simulink model "sensor_correction"  (R2015b)
settings: Solver=FixedStepAuto  StartTime=0.0  StopTime=100  FixedStep=0.001  RelTol=1e-3
libraries: simulink x1
settings Model: Creator=Aleksandar  LastModifiedBy=Aleksandar

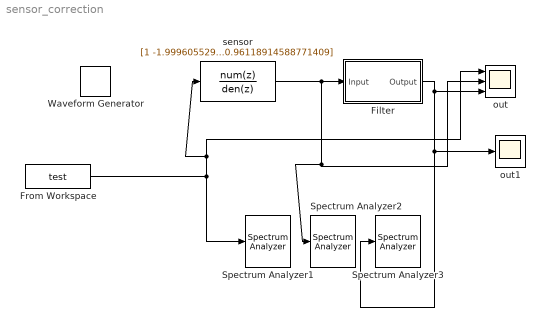
== system sensor_correction ==
  Filter : Subsystem  Tag=FilterWizardSubSystem
      settings: ErrorFcn=dspFilterRealizedInBasicElemsAlgLoopErrFcnCallback
  From Workspace : FromWorkspace  VariableName=test  Interpolate=off  OutputAfterFinalValue=Setting to zero
  Spectrum Analyzer1 : SpectrumAnalyzer
  Spectrum Analyzer2 : SpectrumAnalyzer
  Spectrum Analyzer3 : SpectrumAnalyzer
  Waveform Generator : simulink/Sources/Waveform Generator  OutMin=[]  OutMax=[]  OutDataTypeStr=double  SelectedSignal=1  Signals=sin(1,0.01,0)+sin(1,0.0562,0)+sin(1,0.3162,0)+sin(1,1,0)+sin(1,1.7783,0)+sin(1,10,0)  BlockNames=MultiportSwitch_ab6cea2ffcb549c  SampleTime=0.001
  out : Scope  NumInputPorts=3
  out1 : Scope
  sensor : DiscreteFilter  Tag=BlockMethodSubSystem  Numerator=[1 -1.9996055296176776 0.99960552961767746]  Denominator=[1 -1.9604053759263245 0.96118914588771409]  InputProcessing=Columns as channels (frame based)  FilterStructure=Direct form II transposed  SampleTime=0.001  a0EqualsOne=on
  wires:
  sensor/1 -> out/2, Spectrum Analyzer2/1, Filter/1(Input)
  Filter/1(Output) -> out1/1, Spectrum Analyzer3/1, out/3
  From Workspace/1 -> Spectrum Analyzer1/1, out/1, sensor/1

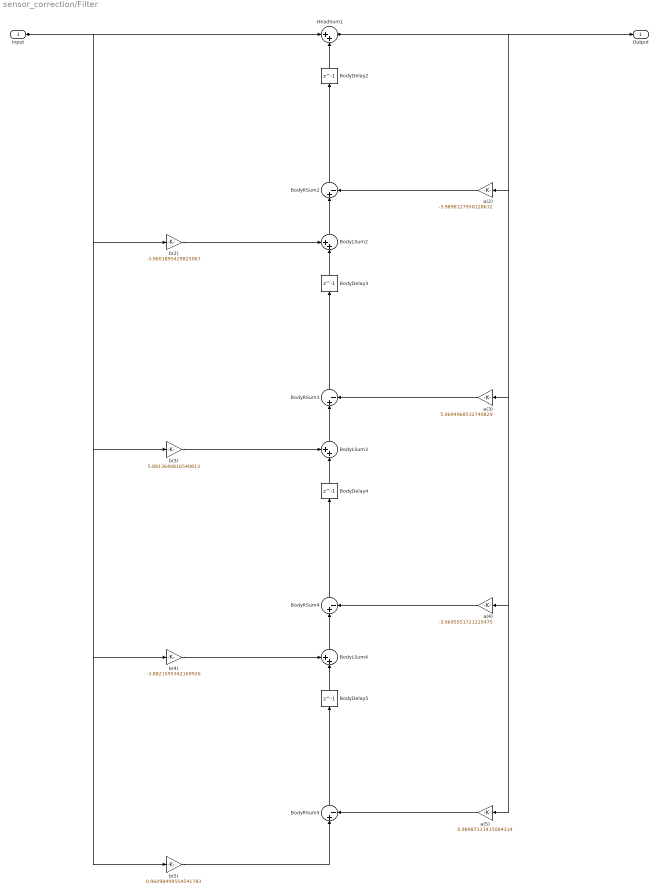
== system sensor_correction/Filter ==
  Input : Inport
  BodyDelay{2..5} (4 alike) : Delay  DelayLength=1  InitialCondition=0
  BodyLSum2 : Sum  Inputs=++|  RndMeth=Nearest  SaturateOnIntegerOverflow=on  OutDataTypeStr=Inherit: Same as first input
  BodyLSum3 : Sum  Inputs=++|  RndMeth=Nearest  SaturateOnIntegerOverflow=on  OutDataTypeStr=Inherit: Same as first input
  BodyLSum4 : Sum  Inputs=++|  RndMeth=Nearest  SaturateOnIntegerOverflow=on  OutDataTypeStr=Inherit: Same as first input
  BodyRSum{2..5} (4 alike) : Sum  Inputs=|+-  RndMeth=Nearest  SaturateOnIntegerOverflow=on  OutDataTypeStr=Inherit: Same as first input
  HeadSum1 : Sum  Inputs=|++  RndMeth=Nearest  SaturateOnIntegerOverflow=on  OutDataTypeStr=Inherit: Same as first input
  a(2) : Gain  Gain=-3.9898127950128632  ParamDataTypeStr=double  RndMeth=Nearest  SaturateOnIntegerOverflow=on  OutDataTypeStr=Inherit: Same as input
  a(3) : Gain  Gain=5.9694968532740829  ParamDataTypeStr=double  RndMeth=Nearest  SaturateOnIntegerOverflow=on  OutDataTypeStr=Inherit: Same as input
  a(4) : Gain  Gain=-3.9695551721225475  ParamDataTypeStr=double  RndMeth=Nearest  SaturateOnIntegerOverflow=on  OutDataTypeStr=Inherit: Same as input
  a(5) : Gain  Gain=0.98987111415004314  ParamDataTypeStr=double  RndMeth=Nearest  SaturateOnIntegerOverflow=on  OutDataTypeStr=Inherit: Same as input
  b(2) : Gain  Gain=-3.9601895429825067  ParamDataTypeStr=double  RndMeth=Nearest  SaturateOnIntegerOverflow=on  OutDataTypeStr=Inherit: Same as input
  b(3) : Gain  Gain=5.8813640816540813  ParamDataTypeStr=double  RndMeth=Nearest  SaturateOnIntegerOverflow=on  OutDataTypeStr=Inherit: Same as input
  b(4) : Gain  Gain=-3.8821595342169926  ParamDataTypeStr=double  RndMeth=Nearest  SaturateOnIntegerOverflow=on  OutDataTypeStr=Inherit: Same as input
  b(5) : Gain  Gain=0.96098499554541783  ParamDataTypeStr=double  RndMeth=Nearest  SaturateOnIntegerOverflow=on  OutDataTypeStr=Inherit: Same as input
  Output : Outport
  wires:
  Input/1 -> HeadSum1/1, b(2)/1, b(3)/1, b(4)/1, b(5)/1
  HeadSum1/1 -> Output/1, a(2)/1, a(3)/1, a(4)/1, a(5)/1
  b(2)/1 -> BodyLSum2/1
  BodyLSum2/1 -> BodyRSum2/1
  BodyRSum2/1 -> BodyDelay2/1
  a(2)/1 -> BodyRSum2/2
  BodyDelay2/1 -> HeadSum1/2
  b(3)/1 -> BodyLSum3/1
  BodyLSum3/1 -> BodyRSum3/1
  BodyRSum3/1 -> BodyDelay3/1
  a(3)/1 -> BodyRSum3/2
  BodyDelay3/1 -> BodyLSum2/2
  b(4)/1 -> BodyLSum4/1
  BodyLSum4/1 -> BodyRSum4/1
  BodyRSum4/1 -> BodyDelay4/1
  a(4)/1 -> BodyRSum4/2
  BodyDelay4/1 -> BodyLSum3/2
  b(5)/1 -> BodyRSum5/1
  BodyRSum5/1 -> BodyDelay5/1
  a(5)/1 -> BodyRSum5/2
  BodyDelay5/1 -> BodyLSum4/2
